simulink model "ex2_model"  (R2024b)
settings: Solver=VariableStepAuto  StartTime=0.0  StopTime=10.0  MaxStep=1e-4  RelTol=1e-3
values from neighbouring files (symbols this model uses):
  A = [0,1; -3, -60]    [ex2_direct.m]
  B = [0; 1]    [ex2_direct.m]
  C = [90, 0]    [ex2_direct.m]
  D = 0    [ex2_direct.m]
  gammao = [gamma(2) - Ld*gamma(1), phio*Ld + phi(2,1) - phi(1,1)*Ld]    [ex2_direct.m]
  Ho = [0; 1]    [ex2_direct.m]
  Jo = [0,1; 0,Ld]    [ex2_direct.m]
  K_robust = Ke(2:end)    [ex2_direct.m]
  Ki = Ke(1)    [ex2_direct.m]
  Nu = feedforward_gains(3)    [ex2_direct.m]
  Nx = feedforward_gains(1:2)    [ex2_direct.m]
  phio = phi(2,2)-Ld*phi(1,2)    [ex2_direct.m]
  ts = 0.001    [ex2_direct.m]
undefined symbols (not defined in the file or in its folder): DiscIntNeverNeededParam, gamma, H, J, phi
settings Model: Creator=Nihal  LastModifiedBy=Nihal

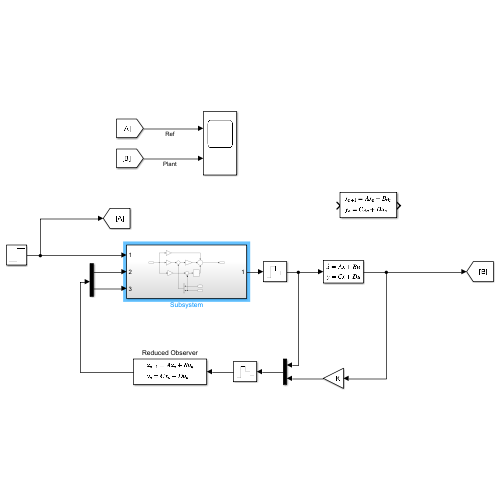
[thumbnail: Simulink's stored preview of the top-level diagram]
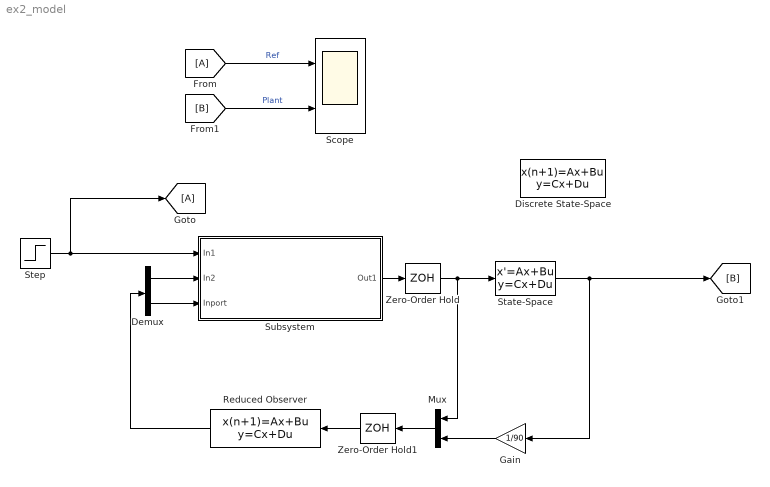
== system ex2_model ==
  Demux : Demux  Outputs=2
  Discrete State-Space : DiscreteStateSpace  A=phi  B=gamma  C=H  D=J  SampleTime=-1
  From : From
  Gain : Gain  Gain=1/90
  Goto : Goto
  Mux : Mux  Inputs=2
  Reduced Observer : DiscreteStateSpace  A=phio  B=gammao  C=Ho  D=Jo  SampleTime=ts
  Scope : Scope  NumInputPorts=2
  State-Space : StateSpace  A=A  B=B  C=C  D=D  InitialCondition=0
  Step : Step  After=40  SampleTime=0
  Subsystem : Subsystem
  Zero-Order Hold : ZeroOrderHold  SampleTime=-1
  Zero-Order Hold1 : ZeroOrderHold  SampleTime=-1
  wires:
  Demux/1 -> Subsystem/2(In2)
  Demux/2 -> Subsystem/3(Inport)
  Step/1 -> Subsystem/1(In1), Goto/1
  Mux/1 -> Zero-Order Hold1/1
  From/1 -> Scope/1  "Ref"
  [B] -> Scope/2  "Plant"
  Reduced Observer/1 -> Demux/1
  Subsystem/1(Out1) -> Zero-Order Hold/1
  State-Space/1 -> [B], Gain/1
  Zero-Order Hold/1 -> State-Space/1, Mux/1
  Zero-Order Hold1/1 -> Reduced Observer/1
  Gain/1 -> Mux/2

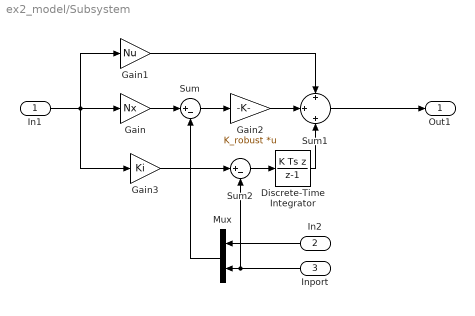
== system ex2_model/Subsystem ==
  In1 : Inport
  In2 : Inport  Port=2
  Inport : Inport  Port=3
  Discrete-Time Integrator : DiscreteIntegrator  IntegratorMethod=Integration: Backward Euler  SampleTime=-1  ICPrevOutput=DiscIntNeverNeededParam  ICPrevScaledInput=DiscIntNeverNeededParam
  Gain : Gain  Gain=Nx
  Gain1 : Gain  Gain=Nu
  Gain2 : Gain  Gain=K_robust  Multiplication=Matrix(K*u)
  Gain3 : Gain  Gain=Ki
  Mux : Mux  Inputs=2
  Sum : Sum  Inputs=|+-
  Sum1 : Sum  Inputs=+|+|+
  Sum2 : Sum  Inputs=|+-
  Out1 : Outport
  wires:
  In1/1 -> Gain3/1, Gain1/1, Gain/1
  Gain/1 -> Sum/1
  Mux/1 -> Sum/2
  Sum/1 -> Gain2/1
  Gain2/1 -> Sum1/2
  Gain1/1 -> Sum1/1
  Sum1/1 -> Out1/1
  In2/1 -> Mux/1
  Inport/1 -> Sum2/2, Mux/2
  Discrete-Time Integrator/1 -> Sum1/3
  Sum2/1 -> Discrete-Time Integrator/1
  Gain3/1 -> Sum2/1
